simulink model "MPCcontrol"  (R2015b)
settings: Solver=FixedStepAuto  StartTime=0.0  StopTime=30  FixedStep=0.01  MaxStep=0.005  RelTol=1e-3
InitFcn:
  | Ts=0.01;
  | dPL22 = 2*dPL2;
values from neighbouring files (symbols this model uses):
  A = [-1/Tg1     0      -1/(R1*Tg1)   0       0       0        0 ... (first row only)    [ObserverModel_2area.m]
  B = [ 1/Tg1 0    0    0 ... (first row only)    [ObserverModel_2area.m]
  C = [0 0 B1  1 0 0 0 ... (first row only)    [ObserverModel_2area.m]
  dPL1 = 0.    (= 0)    [ObserverModel_2area.m]
  dPL2 = 0.1    [ObserverModel_2area.m]
  L = place(A',C',Pole_obs)'    [ObserverModel_2area.m]
settings Model: ModifiedByFormat=Majidi  Creator=Majidi  LastModifiedBy=Majidi
settings DataIOCC: SaveFormat=Array
settings OptimizationCC: ExpressionDepthLimit=2147483647
settings DebuggingCC: UnderspecifiedInitializationDetection=Classic  MergeDetectMultiDrivingBlocksExec=none  SolverPrmCheckMsg=warning  StateNameClashWarn=warning
settings HardwareCC: ProdBitPerPointer=32  ProdLargestAtomicFloat=None  ProdIntDivRoundTo=Undefined  ProdEndianess=Unspecified  ProdWordSize=32  ProdHWDeviceType=32-bit Generic
settings GRTTargetCC: GeneratePreprocessorConditionals=Disable all
settings ConfigComp: CovModelRefEnable=Off

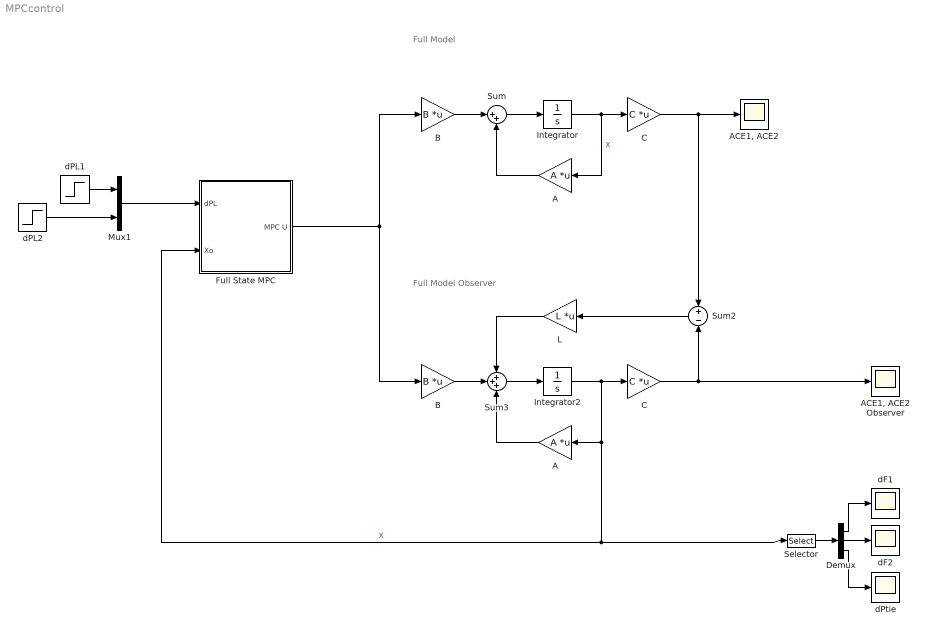
== system MPCcontrol ==
  note: Full Model
  note: Full Model Observer
  A : Gain  Gain=A  Multiplication=Matrix(K*u)
  "A " : Gain  Gain=A  Multiplication=Matrix(K*u)
  "ACE1, ACE2" : Scope
  "ACE1, ACE2 Observer" : Scope
  B : Gain  Gain=B  Multiplication=Matrix(K*u)
  "B " : Gain  Gain=B  Multiplication=Matrix(K*u)
  C : Gain  Gain=C  Multiplication=Matrix(K*u)
  "C " : Gain  Gain=C  Multiplication=Matrix(K*u)
  Demux : Demux  Outputs=3
  Full State MPC : Subsystem
  Integrator : Integrator
  Integrator2 : Integrator
  L : Gain  Gain=L  Multiplication=Matrix(K*u)
  Mux1 : Mux  Inputs=2
  Selector : Selector  InputPortWidth=7  IndexOptions=Index vector (dialog)  Indices=[3 7 4]  OutputSizes=1
  Sum : Sum  Inputs=|++
  Sum2 : Sum  Inputs=+|-
  Sum3 : Sum  Inputs=+++
  dF1 : Scope
  dF2 : Scope
  dPL1 : Step  After=dPL1  SampleTime=0
  dPL2 : Step  After=dPL22  SampleTime=0
  dPtie : Scope
  wires:
  B/1 -> Sum/1
  Sum/1 -> Integrator/1
  A/1 -> Sum/2
  Integrator/1 -> A/1, C/1  "X"
  C/1 -> "ACE1, ACE2"/1, Sum2/1
  dPL1/1 -> Mux1/1
  dPL2/1 -> Mux1/2
  Demux/1 -> dF1/1
  Demux/2 -> dF2/1
  Demux/3 -> dPtie/1
  Selector/1 -> Demux/1
  "B "/1 -> Sum3/2
  Sum3/1 -> Integrator2/1
  "A "/1 -> Sum3/3
  Integrator2/1 -> "C "/1, Full State MPC/2(Xo), Selector/1, "A "/1  "X"
  "C "/1 -> "ACE1, ACE2 Observer"/1, Sum2/2
  Sum2/1 -> L/1
  L/1 -> Sum3/1
  Mux1/1 -> Full State MPC/1(dPL)
  Full State MPC/1(MPC U) -> "B "/1, B/1

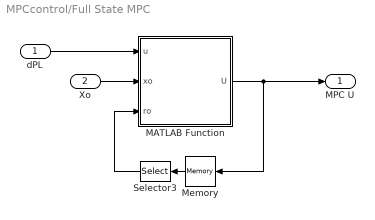
== system MPCcontrol/Full State MPC ==
  dPL : Inport
  Xo : Inport  Port=2
  MATLAB Function : MATLAB Function  TreatAsAtomicUnit=on
  Memory : Memory  X0=[0;0;0;0]
  Selector3 : Selector  InputPortWidth=4  IndexOptions=Index vector (dialog)  Indices=[1 2]  OutputSizes=1
  MPC U : Outport
  wires:
  Memory/1 -> Selector3/1
  Xo/1 -> MATLAB Function/2(xo)
  MATLAB Function/1(U) -> Memory/1, MPC U/1
  dPL/1 -> MATLAB Function/1(u)
  Selector3/1 -> MATLAB Function/3(ro)

== matlab function MPCcontrol/Full State MPC/MATLAB Function ==
  data: u input; U output; xo input; ro input
function U = MPC(u,xo,ro)

% a = [-0.183721545006828,4.21561257448810,0.0114058405037626,0.00367408750026667,-0.236392568501128;-4.16205267369347,-0.0928706956510741,0.0121896199192519,-0.0243240089165755,0.178617279204259;0.0280289737334991,0.0167588644921035,-0.929929171517785,2.13024013261600,-0.0116349231223944;0.00211143008157946,0.0262265264472104,-1.58644954834535,-1.05975076357643,0.105825687137950;-0.00295769226235298,-0.151880268825995,0.00535290487942043,0.0829242254444511,-1.94302936634756];
% b = [0.119647093263081,-0.119204132237909,1.38884507042047,-1.09514401110261;-0.748458880855902,0.549473893827396,0.624028370981700,-0.517316930291258;0.451632878925756,0.494122210734015,-0.992566756213384,-1.02935989327374;0.842051620505800,0.806490112069918,-0.00193123605376590,0.0204784281794829;-0.835488561740107,0.765264017214529,0.122997062160711,-0.114669386020992];
% c = [-1.34792186249645,0.840223590308015,1.08531793877867,-0.745584512522879,-0.825863541107890;1.15752440119341,-0.901756501931565,1.14672775481068,-0.896662736396695,0.793660449878414];
% d = [0,0,0,0;0,0,0,0];

A = [-12.5000000000000,0,-4.16666666666667,0,0,0,0;2.50000000000000,-2.50000000000000,0,0,0,0,0;0,5.99880023995201,-0.0899820035992801,-5.99880023995201,0,0,0;0,0,1.25600000000000,0,0,0,-1.25600000000000;0,0,0,0,-12.5000000000000,0,-4.57875457875458;0,0,0,0,2.27272727272727,-2.27272727272727,0;0,0,0,4.95785820525533,0,4.95785820525533,-0.0793257312840853];
B = [12.5000000000000,0,0,0;0,0,0,0;0,0,-5.99880023995201,0;0,0,0,0;0,12.5000000000000,0,0;0,0,0,0;0,0,0,-4.95785820525533];
C = [0,0,0.425000000000000,1,0,0,0;0,0,0,-1,0,0,0.425000000000000];




yo = C*xo;  

Np = 15;h=0.01;
r = -0.25:h:0.25;
Y1 = zeros(length(r),length(r));Y2=Y1;
y=zeros(2,1);

tol = 1e-5;Ts = 0.01;
if max(abs(yo)) <= tol
    U = [ro;u];
else
    
    
for i=1:length(r)
    Pc1 = r(i);
    for j=1:length(r)
        Pc2 = r(j);
        x=xo;
        for co=1:Np
            X = x+Ts*(A*x+B*[Pc1;Pc2;u]);
            y = C*X;
            x=X;
        end
        Y1(i,j) = y(1);
        Y2(i,j) = y(2);
    end
end
err = abs(Y1)+abs(Y2);
[~,index]=min(err(:));
cul=ceil(index/length(err));
row=floor((index/length(err)-floor(index/length(err)))*length(err));
if row==0
    row=length(err);
end

U = [r(row);r(cul);u];
end
end
